simulink model "IEEE14_case"  (R2024b)
settings: Solver=FixedStepAuto  StartTime=0  StopTime=2  FixedStep=1e-7  RelTol=1e-3
values from neighbouring files (symbols this model uses):
  GFL_15_Bva = 0.009    [IEEE14_parameters.m]
  GFL_15_C_bus_pu = 7.179419    [IEEE14_parameters.m]
  GFL_15_f0 = 60    [IEEE14_parameters.m]
  GFL_15_I_id = 691.26967    [IEEE14_parameters.m]
  GFL_15_I_iq = 691.26967    [IEEE14_parameters.m]
  GFL_15_I_od = 45.2207    [IEEE14_parameters.m]
  GFL_15_I_oq = 45.2207    [IEEE14_parameters.m]
  GFL_15_I_pll = 0.78    [IEEE14_parameters.m]
  GFL_15_Kdi = 0.09    [IEEE14_parameters.m]
  GFL_15_Kdo = 0.9    [IEEE14_parameters.m]
  GFL_15_Kqi = 0.09    [IEEE14_parameters.m]
  GFL_15_Kqo = 0.9    [IEEE14_parameters.m]
  GFL_15_Lg_pu = 0.631447    [IEEE14_parameters.m]
  GFL_15_mode = 1    [IEEE14_parameters.m]
  GFL_15_P_id = 3.7166    [IEEE14_parameters.m]
  GFL_15_P_iq = 3.7166    [IEEE14_parameters.m]
  GFL_15_P_od = 0.4798    [IEEE14_parameters.m]
  GFL_15_P_oq = 0.4798    [IEEE14_parameters.m]
  GFL_15_P_pll = 290.42    [IEEE14_parameters.m]
  GFL_15_Qe_ref = 0.2    [IEEE14_parameters.m]
  GFL_15_Rg_pu = 0.024016    [IEEE14_parameters.m]
  GFL_15_Sbase = 1.000000e+4    (= 10000)    [IEEE14_parameters.m]
  GFL_15_Tdi = 0.01    [IEEE14_parameters.m]
  GFL_15_Tdo = 0.2    [IEEE14_parameters.m]
  GFL_15_Tqi = 0.01    [IEEE14_parameters.m]
  GFL_15_Tqo = 0.2    [IEEE14_parameters.m]
  GFL_15_Vbase = 380    [IEEE14_parameters.m]
  GFL_15_Vdc_ref = 1.011475    [IEEE14_parameters.m]
  GFL_15_Vdcbase = 700    [IEEE14_parameters.m]
  GFL_15_vq_ref = 0    [IEEE14_parameters.m]
  GFL_16_Bva = 0.002    [IEEE14_parameters.m]
  GFL_16_C_bus_pu = 7.179419    [IEEE14_parameters.m]
  GFL_16_f0 = 60    [IEEE14_parameters.m]
  GFL_16_I_id = 691.26967    [IEEE14_parameters.m]
  GFL_16_I_iq = 691.26967    [IEEE14_parameters.m]
  GFL_16_I_od = 45.2207    [IEEE14_parameters.m]
  GFL_16_I_oq = 45.2207    [IEEE14_parameters.m]
  GFL_16_I_pll = 0.78    [IEEE14_parameters.m]
  GFL_16_Kdi = 0.05    [IEEE14_parameters.m]
  GFL_16_Kdo = 0.5    [IEEE14_parameters.m]
  GFL_16_Kqi = 0.05    [IEEE14_parameters.m]
  GFL_16_Kqo = 0.5    [IEEE14_parameters.m]
  GFL_16_Lg_pu = 0.631447    [IEEE14_parameters.m]
  GFL_16_mode = 1    [IEEE14_parameters.m]
  GFL_16_P_id = 3.7166    [IEEE14_parameters.m]
  GFL_16_P_iq = 3.7166    [IEEE14_parameters.m]
  GFL_16_P_od = 0.4798    [IEEE14_parameters.m]
  GFL_16_P_oq = 0.4798    [IEEE14_parameters.m]
  GFL_16_P_pll = 290.42    [IEEE14_parameters.m]
  GFL_16_Qe_ref = 0.2    [IEEE14_parameters.m]
  GFL_16_Rg_pu = 0.024016    [IEEE14_parameters.m]
  GFL_16_Sbase = 1.000000e+4    (= 10000)    [IEEE14_parameters.m]
  GFL_16_Tdi = 0.01    [IEEE14_parameters.m]
  GFL_16_Tdo = 0.2    [IEEE14_parameters.m]
  GFL_16_Tqi = 0.01    [IEEE14_parameters.m]
  GFL_16_Tqo = 0.2    [IEEE14_parameters.m]
  GFL_16_Vbase = 380    [IEEE14_parameters.m]
  GFL_16_Vdc_ref = 1.01144    [IEEE14_parameters.m]
  GFL_16_Vdcbase = 700    [IEEE14_parameters.m]
  GFL_16_vq_ref = 0    [IEEE14_parameters.m]
  GFL_17_Bva = 0.002    [IEEE14_parameters.m]
  GFL_17_C_bus_pu = 7.179419    [IEEE14_parameters.m]
  GFL_17_f0 = 60    [IEEE14_parameters.m]
  GFL_17_I_id = 691.26967    [IEEE14_parameters.m]
  GFL_17_I_iq = 691.26967    [IEEE14_parameters.m]
  GFL_17_I_od = 45.2207    [IEEE14_parameters.m]
  GFL_17_I_oq = 45.2207    [IEEE14_parameters.m]
  GFL_17_I_pll = 0.78    [IEEE14_parameters.m]
  GFL_17_Kdi = 0.05    [IEEE14_parameters.m]
  GFL_17_Kdo = 0.5    [IEEE14_parameters.m]
  GFL_17_Kqi = 0.05    [IEEE14_parameters.m]
  GFL_17_Kqo = 0.5    [IEEE14_parameters.m]
  GFL_17_Lg_pu = 0.631447    [IEEE14_parameters.m]
  GFL_17_mode = 1    [IEEE14_parameters.m]
  GFL_17_P_id = 3.7166    [IEEE14_parameters.m]
  GFL_17_P_iq = 3.7166    [IEEE14_parameters.m]
  GFL_17_P_od = 0.4798    [IEEE14_parameters.m]
  GFL_17_P_oq = 0.4798    [IEEE14_parameters.m]
  GFL_17_P_pll = 290.42    [IEEE14_parameters.m]
  GFL_17_Qe_ref = 0.2    [IEEE14_parameters.m]
  GFL_17_Rg_pu = 0.024016    [IEEE14_parameters.m]
  GFL_17_Sbase = 1.000000e+4    (= 10000)    [IEEE14_parameters.m]
  GFL_17_Tdi = 0.01    [IEEE14_parameters.m]
  GFL_17_Tdo = 0.2    [IEEE14_parameters.m]
  GFL_17_Tqi = 0.01    [IEEE14_parameters.m]
  GFL_17_Tqo = 0.2    [IEEE14_parameters.m]
  GFL_17_Vbase = 380    [IEEE14_parameters.m]
  GFL_17_Vdc_ref = 1.011632    [IEEE14_parameters.m]
  GFL_17_Vdcbase = 700    [IEEE14_parameters.m]
  GFL_17_vq_ref = 0    [IEEE14_parameters.m]
  GFL_18_Bva = 0.002    [IEEE14_parameters.m]
  GFL_18_C_bus_pu = 7.179419    [IEEE14_parameters.m]
  GFL_18_f0 = 60    [IEEE14_parameters.m]
  GFL_18_I_id = 691.26967    [IEEE14_parameters.m]
  GFL_18_I_iq = 691.26967    [IEEE14_parameters.m]
  GFL_18_I_od = 45.2207    [IEEE14_parameters.m]
  GFL_18_I_oq = 45.2207    [IEEE14_parameters.m]
  GFL_18_I_pll = 0.78    [IEEE14_parameters.m]
  GFL_18_Kdi = 0.05    [IEEE14_parameters.m]
  GFL_18_Kdo = 0.5    [IEEE14_parameters.m]
  GFL_18_Kqi = 0.05    [IEEE14_parameters.m]
  GFL_18_Kqo = 0.5    [IEEE14_parameters.m]
  GFL_18_Lg_pu = 0.631447    [IEEE14_parameters.m]
  GFL_18_mode = 1    [IEEE14_parameters.m]
  GFL_18_P_id = 3.7166    [IEEE14_parameters.m]
  GFL_18_P_iq = 3.7166    [IEEE14_parameters.m]
  GFL_18_P_od = 0.4798    [IEEE14_parameters.m]
  GFL_18_P_oq = 0.4798    [IEEE14_parameters.m]
  GFL_18_P_pll = 290.42    [IEEE14_parameters.m]
  GFL_18_Qe_ref = 0.2    [IEEE14_parameters.m]
  GFL_18_Rg_pu = 0.024016    [IEEE14_parameters.m]
  GFL_18_Sbase = 1.000000e+4    (= 10000)    [IEEE14_parameters.m]
  GFL_18_Tdi = 0.01    [IEEE14_parameters.m]
  GFL_18_Tdo = 0.2    [IEEE14_parameters.m]
  GFL_18_Tqi = 0.01    [IEEE14_parameters.m]
  GFL_18_Tqo = 0.2    [IEEE14_parameters.m]
  GFL_18_Vbase = 380    [IEEE14_parameters.m]
  GFL_18_Vdc_ref = 1.011572    [IEEE14_parameters.m]
  GFL_18_Vdcbase = 700    [IEEE14_parameters.m]
  GFL_18_vq_ref = 0    [IEEE14_parameters.m]
  ... (+180 more)
(part 2 of 25)

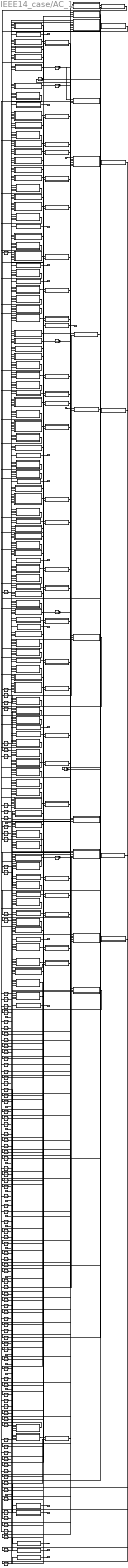
== system IEEE14_case/AC_1 ==
  id_SG_D_1 : Inport
  iq_SG_D_1 : Inport  Port=2
  id_SG_D_2 : Inport  Port=3
  iq_SG_D_2 : Inport  Port=4
  id_SG_D_3 : Inport  Port=5
  iq_SG_D_3 : Inport  Port=6
  id_SG_D_6 : Inport  Port=7
  iq_SG_D_6 : Inport  Port=8
  id_SG_D_8 : Inport  Port=9
  iq_SG_D_8 : Inport  Port=10
  id_GFL_15 : Inport  Port=11
  iq_GFL_15 : Inport  Port=12
  id_GFL_16 : Inport  Port=13
  iq_GFL_16 : Inport  Port=14
  id_GFL_17 : Inport  Port=15
  iq_GFL_17 : Inport  Port=16
  id_GFL_18 : Inport  Port=17
  iq_GFL_18 : Inport  Port=18
  d_id_line_10_11_block : Subsystem
  d_id_line_11_15_block : Subsystem
  d_id_line_12_13_block : Subsystem
  d_id_line_12_16_block : Subsystem
  d_id_line_13_14_block : Subsystem
  d_id_line_13_17_block : Subsystem
  d_id_line_14_18_block : Subsystem
  d_id_line_1_2_block : Subsystem
  d_id_line_1_5_block : Subsystem
  d_id_line_2_3_block : Subsystem
  d_id_line_2_4_block : Subsystem
  d_id_line_2_5_block : Subsystem
  d_id_line_3_4_block : Subsystem
  d_id_line_4_5_block : Subsystem
  d_id_line_4_7_block : Subsystem
  d_id_line_4_9_block : Subsystem
  d_id_line_5_6_block : Subsystem
  d_id_line_6_11_block : Subsystem
  d_id_line_6_12_block : Subsystem
  d_id_line_6_13_block : Subsystem
  d_id_line_7_8_block : Subsystem
  d_id_line_7_9_block : Subsystem
  d_id_line_9_10_block : Subsystem
  d_id_line_9_14_block : Subsystem
  d_id_load_10_block : Subsystem
  d_id_load_11_block : Subsystem
  d_id_load_12_block : Subsystem
  d_id_load_13_block : Subsystem
  d_id_load_14_block : Subsystem
  d_id_load_2_block : Subsystem
  d_id_load_3_block : Subsystem
  d_id_load_4_block : Subsystem
  d_id_load_5_block : Subsystem
  d_id_load_6_block : Subsystem
  d_id_load_9_block : Subsystem
  d_iq_line_10_11_block : Subsystem
  d_iq_line_11_15_block : Subsystem
  d_iq_line_12_13_block : Subsystem
  d_iq_line_12_16_block : Subsystem
  d_iq_line_13_14_block : Subsystem
  d_iq_line_13_17_block : Subsystem
  d_iq_line_14_18_block : Subsystem
  d_iq_line_1_2_block : Subsystem
  d_iq_line_1_5_block : Subsystem
  d_iq_line_2_3_block : Subsystem
  d_iq_line_2_4_block : Subsystem
  d_iq_line_2_5_block : Subsystem
  d_iq_line_3_4_block : Subsystem
  d_iq_line_4_5_block : Subsystem
  d_iq_line_4_7_block : Subsystem
  d_iq_line_4_9_block : Subsystem
  d_iq_line_5_6_block : Subsystem
  d_iq_line_6_11_block : Subsystem
  d_iq_line_6_12_block : Subsystem
  d_iq_line_6_13_block : Subsystem
  d_iq_line_7_8_block : Subsystem
  d_iq_line_7_9_block : Subsystem
  d_iq_line_9_10_block : Subsystem
  d_iq_line_9_14_block : Subsystem
  d_iq_load_10_block : Subsystem
  d_iq_load_11_block : Subsystem
  d_iq_load_12_block : Subsystem
  d_iq_load_13_block : Subsystem
  d_iq_load_14_block : Subsystem
  d_iq_load_2_block : Subsystem
  d_iq_load_3_block : Subsystem
  d_iq_load_4_block : Subsystem
  d_iq_load_5_block : Subsystem
  d_iq_load_6_block : Subsystem
  d_iq_load_9_block : Subsystem
  d_vd_bus_10_block : Subsystem
  d_vd_bus_11_block : Subsystem
  d_vd_bus_12_block : Subsystem
  d_vd_bus_13_block : Subsystem
  d_vd_bus_14_block : Subsystem
  d_vd_bus_15_block : Subsystem
  d_vd_bus_16_block : Subsystem
  d_vd_bus_17_block : Subsystem
  d_vd_bus_18_block : Subsystem
  d_vd_bus_1_block : Subsystem
  d_vd_bus_2_block : Subsystem
  d_vd_bus_3_block : Subsystem
  d_vd_bus_4_block : Subsystem
  d_vd_bus_5_block : Subsystem
  d_vd_bus_6_block : Subsystem
  d_vd_bus_7_block : Subsystem
  d_vd_bus_8_block : Subsystem
  d_vd_bus_9_block : Subsystem
  d_vq_bus_10_block : Subsystem
  d_vq_bus_11_block : Subsystem
  d_vq_bus_12_block : Subsystem
  d_vq_bus_13_block : Subsystem
  d_vq_bus_14_block : Subsystem
  d_vq_bus_15_block : Subsystem
  d_vq_bus_16_block : Subsystem
  d_vq_bus_17_block : Subsystem
  d_vq_bus_18_block : Subsystem
  d_vq_bus_1_block : Subsystem
  d_vq_bus_2_block : Subsystem
  d_vq_bus_3_block : Subsystem
  d_vq_bus_4_block : Subsystem
  d_vq_bus_5_block : Subsystem
  d_vq_bus_6_block : Subsystem
  d_vq_bus_7_block : Subsystem
  d_vq_bus_8_block : Subsystem
  d_vq_bus_9_block : Subsystem
  id_bus_10_block : Subsystem
  id_bus_11_block : Subsystem
  id_bus_12_block : Subsystem
  id_bus_13_block : Subsystem
  id_bus_14_block : Subsystem
  id_bus_15_block : Subsystem
  id_bus_16_block : Subsystem
  id_bus_17_block : Subsystem
  id_bus_18_block : Subsystem
  id_bus_1_block : Subsystem
  id_bus_2_block : Subsystem
  id_bus_3_block : Subsystem
  id_bus_4_block : Subsystem
  id_bus_5_block : Subsystem
  id_bus_6_block : Subsystem
  id_bus_7_block : Subsystem
  id_bus_8_block : Subsystem
  id_bus_9_block : Subsystem
  id_line_10_11 : Integrator  InitialCondition=-0.0994
  id_line_11_15 : Integrator  InitialCondition=-0.0847
  id_line_12_13 : Integrator  InitialCondition=0.0298
  id_line_12_16 : Integrator  InitialCondition=-0.0848
  id_line_13_14 : Integrator  InitialCondition=0.0471
  id_line_13_17 : Integrator  InitialCondition=-0.0854
  id_line_14_18 : Integrator  InitialCondition=-0.0844
  id_line_1_2 : Integrator  InitialCondition=1.2072
  id_line_1_5 : Integrator  InitialCondition=0.5833
  id_line_2_3 : Integrator  InitialCondition=0.6304
  id_line_2_4 : Integrator  InitialCondition=0.4483
  id_line_2_5 : Integrator  InitialCondition=0.3091
  id_line_3_4 : Integrator  InitialCondition=-0.2633
  id_line_4_5 : Integrator  InitialCondition=-0.6044
  id_line_4_7 : Integrator  InitialCondition=0.2064
  id_line_4_9 : Integrator  InitialCondition=0.1163
  id_line_5_6 : Integrator  InitialCondition=0.1823
  id_line_6_11 : Integrator  InitialCondition=0.0515
  id_line_6_12 : Integrator  InitialCondition=0.0172
  id_line_6_13 : Integrator  InitialCondition=0.0733
  id_line_7_8 : Integrator  InitialCondition=-0.0016
  id_line_7_9 : Integrator  InitialCondition=0.1862
  id_line_9_10 : Integrator  InitialCondition=0.0183
  id_line_9_14 : Integrator  InitialCondition=-0.0029
  id_load_10 : Integrator  InitialCondition=0.06873535659071953
  id_load_11 : Integrator  InitialCondition=0.028343117438752577
  id_load_12 : Integrator  InitialCondition=0.05203066731118701
  id_load_13 : Integrator  InitialCondition=0.11216160588057182
  id_load_14 : Integrator  InitialCondition=0.12451829566194553
  id_load_2 : Integrator  InitialCondition=0.19861496427307673
  id_load_3 : Integrator  InitialCondition=0.8795187658248551
  id_load_4 : Integrator  InitialCondition=0.4432908881339787
  id_load_5 : Integrator  InitialCondition=0.06927735163817465
  id_load_6 : Integrator  InitialCondition=0.09154605340717285
  id_load_9 : Integrator  InitialCondition=0.23186808645820936
  iq_bus_10_block : Subsystem
  iq_bus_11_block : Subsystem
  iq_bus_12_block : Subsystem
  iq_bus_13_block : Subsystem
  iq_bus_14_block : Subsystem
  iq_bus_15_block : Subsystem
  iq_bus_16_block : Subsystem
  iq_bus_17_block : Subsystem
  iq_bus_18_block : Subsystem
  iq_bus_1_block : Subsystem
  iq_bus_2_block : Subsystem
  iq_bus_3_block : Subsystem
  iq_bus_4_block : Subsystem
  iq_bus_5_block : Subsystem
  iq_bus_6_block : Subsystem
  iq_bus_7_block : Subsystem
  iq_bus_8_block : Subsystem
  iq_bus_9_block : Subsystem
  iq_line_10_11 : Integrator  InitialCondition=-0.0778
  iq_line_11_15 : Integrator  InitialCondition=0.0403
  iq_line_12_13 : Integrator  InitialCondition=-0.0166
  iq_line_12_16 : Integrator  InitialCondition=0.0398
  iq_line_13_14 : Integrator  InitialCondition=0.0205
  iq_line_13_17 : Integrator  InitialCondition=0.0402
  iq_line_14_18 : Integrator  InitialCondition=0.0417
  iq_line_1_2 : Integrator  InitialCondition=0.0983
  iq_line_1_5 : Integrator  InitialCondition=0.0958
  iq_line_2_3 : Integrator  InitialCondition=-0.1082
  iq_line_2_4 : Integrator  InitialCondition=0.1344
  iq_line_2_5 : Integrator  InitialCondition=0.1439
  iq_line_3_4 : Integrator  InitialCondition=0.1816
  iq_line_4_5 : Integrator  InitialCondition=0.0405
  iq_line_4_7 : Integrator  InitialCondition=0.1587
  iq_line_4_9 : Integrator  InitialCondition=0.0708
  iq_line_5_6 : Integrator  InitialCondition=0.0222
  iq_line_6_11 : Integrator  InitialCondition=0.1413
  iq_line_6_12 : Integrator  InitialCondition=0.11
  iq_line_6_13 : Integrator  InitialCondition=0.1609
  iq_line_7_8 : Integrator  InitialCondition=-0.0082
  iq_line_7_9 : Integrator  InitialCondition=0.0516
  iq_line_9_10 : Integrator  InitialCondition=0.0881
  iq_line_9_14 : Integrator  InitialCondition=-0.0308
  iq_load_10 : Integrator  InitialCondition=-0.06784560660059201
  iq_load_11 : Integrator  InitialCondition=-0.021996168279197863
  iq_load_12 : Integrator  InitialCondition=-0.02423326671806508
  iq_load_13 : Integrator  InitialCondition=-0.0749088369050284
  iq_load_14 : Integrator  InitialCondition=-0.07210105053188964
  iq_load_2 : Integrator  InitialCondition=-0.13580394701233528
  iq_load_3 : Integrator  InitialCondition=-0.3629254076686232
  iq_load_4 : Integrator  InitialCondition=-0.10576972487588117
  iq_load_5 : Integrator  InitialCondition=-0.02416665828239703
  iq_load_6 : Integrator  InitialCondition=-0.0865380168455866
  iq_load_9 : Integrator  InitialCondition=-0.20188514867386012
  vd_bus_1 : Integrator  InitialCondition=1.06
  vd_bus_10 : Integrator  InitialCondition=1.0850866003154533
  vd_bus_11 : Integrator  InitialCondition=1.0782933921318274
  vd_bus_12 : Integrator  InitialCondition=1.0810945989476521
  vd_bus_13 : Integrator  InitialCondition=1.0711851912075123
  vd_bus_14 : Integrator  InitialCondition=1.0702741301344978
  vd_bus_15 : Integrator  InitialCondition=1.1116110968480268
  vd_bus_15_out_block : Subsystem
  vd_bus_16 : Integrator  InitialCondition=1.11407591885913
  vd_bus_16_out_block : Subsystem
  vd_bus_17 : Integrator  InitialCondition=1.1044709003041506
  vd_bus_17_out_block : Subsystem
  vd_bus_18 : Integrator  InitialCondition=1.1045577407027038
  vd_bus_18_out_block : Subsystem
  vd_bus_1_out_block : Subsystem
  vd_bus_2 : Integrator  InitialCondition=1.0424236711882215
  vd_bus_2_out_block : Subsystem
  vd_bus_3 : Integrator  InitialCondition=0.9913775753162218
  vd_bus_3_out_block : Subsystem
  vd_bus_4 : Integrator  InitialCondition=1.040078267757068
  vd_bus_5 : Integrator  InitialCondition=1.0498509288179132
  vd_bus_6 : Integrator  InitialCondition=1.055074232738516
  vd_bus_6_out_block : Subsystem
  vd_bus_7 : Integrator  InitialCondition=1.072545462130714
  vd_bus_8 : Integrator  InitialCondition=1.0710963964517566
  vd_bus_8_out_block : Subsystem
  vd_bus_9 : Integrator  InitialCondition=1.0782222211377726
  vq_bus_1 : Integrator  InitialCondition=0.0
  vq_bus_10 : Integrator  InitialCondition=-0.22722452297111975
  vq_bus_11 : Integrator  InitialCondition=-0.2017534916558011
  vq_bus_12 : Integrator  InitialCondition=-0.19600851364759078
  vq_bus_13 : Integrator  InitialCondition=-0.19829634756591635
  vq_bus_14 : Integrator  InitialCondition=-0.21818391422220956
  vq_bus_15 : Integrator  InitialCondition=-0.1448821101871742
  vq_bus_15_out_block : Subsystem
  vq_bus_16 : Integrator  InitialCondition=-0.13904857608995075
  vq_bus_16_out_block : Subsystem
  vq_bus_17 : Integrator  InitialCondition=-0.140924628484122
  vq_bus_17_out_block : Subsystem
  vq_bus_18 : Integrator  InitialCondition=-0.16158890681408472
  vq_bus_18_out_block : Subsystem
  vq_bus_1_out_block : Subsystem
  vq_bus_2 : Integrator  InitialCondition=-0.07333409675226385
  vq_bus_2_out_block : Subsystem
  vq_bus_3 : Integrator  InitialCondition=-0.1930556996312955
  vq_bus_3_out_block : Subsystem
  vq_bus_4 : Integrator  InitialCondition=-0.1601855443701038
  vq_bus_5 : Integrator  InitialCondition=-0.13527348292909663
  vq_bus_6 : Integrator  InitialCondition=-0.17809650027788754
  vq_bus_6_out_block : Subsystem
  vq_bus_7 : Integrator  InitialCondition=-0.20239348167849394
  vq_bus_8 : Integrator  InitialCondition=-0.20212003737398646
  vq_bus_8_out_block : Subsystem
  vq_bus_9 : Integrator  InitialCondition=-0.22287264369679838
  vd_bus_1_out : Outport
  vq_bus_1_out : Outport  Port=2
  vd_bus_2_out : Outport  Port=3
  vq_bus_2_out : Outport  Port=4
  vd_bus_3_out : Outport  Port=5
  vq_bus_3_out : Outport  Port=6
  vd_bus_6_out : Outport  Port=7
  vq_bus_6_out : Outport  Port=8
  vd_bus_8_out : Outport  Port=9
  vq_bus_8_out : Outport  Port=10
  vd_bus_15_out : Outport  Port=11
  vq_bus_15_out : Outport  Port=12
  vd_bus_16_out : Outport  Port=13
  vq_bus_16_out : Outport  Port=14
  vd_bus_17_out : Outport  Port=15
  vq_bus_17_out : Outport  Port=16
  vd_bus_18_out : Outport  Port=17
  vq_bus_18_out : Outport  Port=18
  wires:
  d_id_load_12_block/1(Blockout_d_id_load_12_58f44) -> id_load_12/1
  vd_bus_8/1 -> vd_bus_8_out_block/1(State_vd_bus_8_bc007), d_id_line_7_8_block/3(State_vd_bus_8_dd54f), d_vq_bus_8_block/2(State_vd_bus_8_3801a)
  vq_bus_16_out_block/1(Blockout_vq_bus_16_out_7f446) -> vq_bus_16_out/1
  d_vq_bus_11_block/1(Blockout_d_vq_bus_11_d741b) -> vq_bus_11/1
  id_GFL_15/1 -> id_bus_15_block/1(Input_id_GFL_15_c7559)
  d_id_line_9_14_block/1(Blockout_d_id_line_9_14_6ccdc) -> id_line_9_14/1
  iq_GFL_17/1 -> iq_bus_17_block/1(Input_iq_GFL_17_ce0cb)
  d_id_line_6_12_block/1(Blockout_d_id_line_6_12_9a391) -> id_line_6_12/1
  iq_GFL_18/1 -> iq_bus_18_block/1(Input_iq_GFL_18_ec44c)
  id_line_12_16/1 -> d_id_line_12_16_block/1(State_id_line_12_16_7c285), d_iq_line_12_16_block/1(State_id_line_12_16_8add4), id_bus_16_block/2(State_id_line_12_16_7c95c), id_bus_12_block/4(State_id_line_12_16_716c0)
  iq_bus_6_block/1(Blockout_iq_bus_6_4d630) -> d_vq_bus_6_block/1(Alge_iq_bus_6_86836)
  d_vq_bus_15_block/1(Blockout_d_vq_bus_15_3c6af) -> vq_bus_15/1
  id_load_10/1 -> d_id_load_10_block/1(State_id_load_10_31e9c), d_iq_load_10_block/1(State_id_load_10_0a094), id_bus_10_block/1(State_id_load_10_5dfe0)
  id_line_7_8/1 -> d_iq_line_7_8_block/1(State_id_line_7_8_32461), id_bus_7_block/2(State_id_line_7_8_a9fc4), id_bus_8_block/2(State_id_line_7_8_1f3e4)
  id_SG_D_2/1 -> id_bus_2_block/1(Input_id_SG_D_2_87b72)
  iq_line_4_5/1 -> iq_bus_4_block/4(State_iq_line_4_5_4a221), iq_bus_5_block/4(State_iq_line_4_5_98539), d_id_line_4_5_block/2(State_iq_line_4_5_5f8a8), d_iq_line_4_5_block/2(State_iq_line_4_5_0332d)
  d_id_line_7_9_block/1(Blockout_d_id_line_7_9_bf772) -> id_line_7_9/1
  id_bus_8_block/1(Blockout_id_bus_8_d2e4f) -> d_vd_bus_8_block/1(Alge_id_bus_8_67a63)
  vq_bus_2/1 -> d_vd_bus_2_block/2(State_vq_bus_2_bcae6), d_iq_line_1_2_block/4(State_vq_bus_2_0b7a1), d_iq_line_2_5_block/3(State_vq_bus_2_080ca), d_iq_line_2_4_block/3(State_vq_bus_2_24316), d_iq_load_2_block/3(State_vq_bus_2_25b3a), vq_bus_2_out_block/1(State_vq_bus_2_ea0d1), d_iq_line_2_3_block/3(State_vq_bus_2_4a159)
  id_GFL_18/1 -> id_bus_18_block/1(Input_id_GFL_18_1db57)
  d_vq_bus_12_block/1(Blockout_d_vq_bus_12_08cfc) -> vq_bus_12/1
  id_bus_13_block/1(Blockout_id_bus_13_73688) -> d_vd_bus_13_block/1(Alge_id_bus_13_3078a)
  iq_bus_16_block/1(Blockout_iq_bus_16_71499) -> d_vq_bus_16_block/1(Alge_iq_bus_16_45d99)
  iq_line_12_16/1 -> d_iq_line_12_16_block/2(State_iq_line_12_16_8bc6b), iq_bus_12_block/4(State_iq_line_12_16_8cacc), iq_bus_16_block/2(State_iq_line_12_16_2996d), d_id_line_12_16_block/2(State_iq_line_12_16_b3649)
  d_iq_load_12_block/1(Blockout_d_iq_load_12_9f109) -> iq_load_12/1
  d_iq_line_4_5_block/1(Blockout_d_iq_line_4_5_de0fa) -> iq_line_4_5/1
  d_id_line_10_11_block/1(Blockout_d_id_line_10_11_2eb24) -> id_line_10_11/1
  vd_bus_16_out_block/1(Blockout_vd_bus_16_out_bf920) -> vd_bus_16_out/1
  id_GFL_16/1 -> id_bus_16_block/1(Input_id_GFL_16_67778)
  id_GFL_17/1 -> id_bus_17_block/1(Input_id_GFL_17_1404c)
  vd_bus_14/1 -> d_id_load_14_block/3(State_vd_bus_14_a8c17), d_id_line_14_18_block/3(State_vd_bus_14_f98b2), d_id_line_9_14_block/3(State_vd_bus_14_60cbb), d_vq_bus_14_block/2(State_vd_bus_14_b82c6), d_id_line_13_14_block/4(State_vd_bus_14_db328)
  iq_line_6_11/1 -> iq_bus_6_block/4(State_iq_line_6_11_dc417), iq_bus_11_block/2(State_iq_line_6_11_3bc55), d_id_line_6_11_block/2(State_iq_line_6_11_43c10), d_iq_line_6_11_block/2(State_iq_line_6_11_23688)
  iq_SG_D_3/1 -> iq_bus_3_block/1(Input_iq_SG_D_3_f2caf)
  d_id_load_14_block/1(Blockout_d_id_load_14_efc39) -> id_load_14/1
  id_line_2_3/1 -> id_bus_2_block/4(State_id_line_2_3_47528), id_bus_3_block/3(State_id_line_2_3_0c1e5), d_iq_line_2_3_block/1(State_id_line_2_3_74cbb), d_id_line_2_3_block/1(State_id_line_2_3_bbe6e)
  iq_GFL_15/1 -> iq_bus_15_block/1(Input_iq_GFL_15_581cf)
  iq_GFL_16/1 -> iq_bus_16_block/1(Input_iq_GFL_16_66c6c)
  d_id_line_9_10_block/1(Blockout_d_id_line_9_10_ec156) -> id_line_9_10/1
  vd_bus_4/1 -> d_id_line_2_4_block/4(State_vd_bus_4_3c016), d_id_line_4_5_block/3(State_vd_bus_4_6b1ed), d_id_line_4_7_block/2(State_vd_bus_4_7fac7), d_id_load_4_block/3(State_vd_bus_4_11e1c), d_id_line_4_9_block/2(State_vd_bus_4_34e3c), d_id_line_3_4_block/4(State_vd_bus_4_4b57b), d_vq_bus_4_block/2(State_vd_bus_4_7baed)
  id_bus_18_block/1(Blockout_id_bus_18_37cb9) -> d_vd_bus_18_block/1(Alge_id_bus_18_48e95)
  id_bus_9_block/1(Blockout_id_bus_9_1c066) -> d_vd_bus_9_block/1(Alge_id_bus_9_e9a9d)
  iq_load_9/1 -> d_id_load_9_block/2(State_iq_load_9_3ccc7), iq_bus_9_block/1(State_iq_load_9_b0a53), d_iq_load_9_block/2(State_iq_load_9_3e6fb)
  iq_bus_9_block/1(Blockout_iq_bus_9_d3dd5) -> d_vq_bus_9_block/1(Alge_iq_bus_9_5db18)
  d_iq_line_11_15_block/1(Blockout_d_iq_line_11_15_665a1) -> iq_line_11_15/1
  iq_line_7_8/1 -> iq_bus_8_block/2(State_iq_line_7_8_02a2e), iq_bus_7_block/2(State_iq_line_7_8_54428), d_id_line_7_8_block/1(State_iq_line_7_8_7266b)
  vd_bus_15_out_block/1(Blockout_vd_bus_15_out_53236) -> vd_bus_15_out/1
  vq_bus_18/1 -> d_vd_bus_18_block/2(State_vq_bus_18_c75a6), d_iq_line_14_18_block/4(State_vq_bus_18_e3293), vq_bus_18_out_block/1(State_vq_bus_18_e31db)
  iq_SG_D_6/1 -> iq_bus_6_block/1(Input_iq_SG_D_6_fd9b5)
  iq_SG_D_8/1 -> iq_bus_8_block/1(Input_iq_SG_D_8_05cc5)
  vd_bus_18_out_block/1(Blockout_vd_bus_18_out_c2e2f) -> vd_bus_18_out/1
  id_load_5/1 -> id_bus_5_block/1(State_id_load_5_1b867), d_iq_load_5_block/1(State_id_load_5_e43f2), d_id_load_5_block/1(State_id_load_5_82a6e)
  vq_bus_12/1 -> d_vd_bus_12_block/2(State_vq_bus_12_ee0ac), d_iq_line_12_16_block/3(State_vq_bus_12_58935), d_iq_load_12_block/3(State_vq_bus_12_83802), d_iq_line_12_13_block/3(State_vq_bus_12_5dc3a), d_iq_line_6_12_block/3(State_vq_bus_12_69550)
  id_SG_D_8/1 -> id_bus_8_block/1(Input_id_SG_D_8_15cec)
  d_id_load_11_block/1(Blockout_d_id_load_11_86202) -> id_load_11/1
  vq_bus_17/1 -> d_vd_bus_17_block/2(State_vq_bus_17_647a1), d_iq_line_13_17_block/4(State_vq_bus_17_e9502), vq_bus_17_out_block/1(State_vq_bus_17_ceb31)
  iq_bus_18_block/1(Blockout_iq_bus_18_97ded) -> d_vq_bus_18_block/1(Alge_iq_bus_18_569e7)
  iq_line_6_12/1 -> d_id_line_6_12_block/2(State_iq_line_6_12_68573), iq_bus_6_block/5(State_iq_line_6_12_b02a7), iq_bus_12_block/2(State_iq_line_6_12_a1863), d_iq_line_6_12_block/2(State_iq_line_6_12_950d7)
  id_SG_D_3/1 -> id_bus_3_block/1(Input_id_SG_D_3_ffe04)
  id_SG_D_6/1 -> id_bus_6_block/1(Input_id_SG_D_6_e5cad)
  iq_bus_1_block/1(Blockout_iq_bus_1_352cb) -> d_vq_bus_1_block/1(Alge_iq_bus_1_7f6e6)
  iq_SG_D_2/1 -> iq_bus_2_block/1(Input_iq_SG_D_2_8fd05)
  vd_bus_1/1 -> d_vq_bus_1_block/2(State_vd_bus_1_cd54b), vd_bus_1_out_block/1(State_vd_bus_1_5dc0e), d_id_line_1_5_block/3(State_vd_bus_1_768e4), d_id_line_1_2_block/3(State_vd_bus_1_70d37)
  id_bus_17_block/1(Blockout_id_bus_17_789d1) -> d_vd_bus_17_block/1(Alge_id_bus_17_262b4)
  vq_bus_2_out_block/1(Blockout_vq_bus_2_out_c2eb9) -> vq_bus_2_out/1
  vd_bus_6/1 -> d_vq_bus_6_block/2(State_vd_bus_6_d464c), d_id_load_6_block/3(State_vd_bus_6_858b4), d_id_line_6_12_block/4(State_vd_bus_6_ffde5), d_id_line_6_13_block/4(State_vd_bus_6_845eb), vd_bus_6_out_block/1(State_vd_bus_6_a4f60), d_id_line_5_6_block/3(State_vd_bus_6_a8e09), d_id_line_6_11_block/4(State_vd_bus_6_98960)
  d_vd_bus_18_block/1(Blockout_d_vd_bus_18_49967) -> vd_bus_18/1
  iq_SG_D_1/1 -> iq_bus_1_block/1(Input_iq_SG_D_1_56ece)
  iq_line_2_5/1 -> iq_bus_5_block/3(State_iq_line_2_5_08804), d_id_line_2_5_block/2(State_iq_line_2_5_b0efa), iq_bus_2_block/6(State_iq_line_2_5_fb0c4), d_iq_line_2_5_block/2(State_iq_line_2_5_dd836)
  iq_bus_3_block/1(Blockout_iq_bus_3_60c7d) -> d_vq_bus_3_block/1(Alge_iq_bus_3_8efd3)
  id_SG_D_1/1 -> id_bus_1_block/1(Input_id_SG_D_1_3327d)
  id_bus_1_block/1(Blockout_id_bus_1_ba05b) -> d_vd_bus_1_block/1(Alge_id_bus_1_90b3c)
  vd_bus_7/1 -> d_vq_bus_7_block/2(State_vd_bus_7_1c88a), d_id_line_4_7_block/3(State_vd_bus_7_4017f), d_id_line_7_9_block/2(State_vd_bus_7_8bd9d), d_id_line_7_8_block/2(State_vd_bus_7_8b12e)
  d_vq_bus_4_block/1(Blockout_d_vq_bus_4_75eba) -> vq_bus_4/1
  vd_bus_16/1 -> d_vq_bus_16_block/2(State_vd_bus_16_358d8), d_id_line_12_16_block/4(State_vd_bus_16_b2ca7), vd_bus_16_out_block/1(State_vd_bus_16_c68f5)
  id_bus_5_block/1(Blockout_id_bus_5_9fe33) -> d_vd_bus_5_block/1(Alge_id_bus_5_3a39c)
  iq_line_9_10/1 -> d_id_line_9_10_block/2(State_iq_line_9_10_22e13), d_iq_line_9_10_block/2(State_iq_line_9_10_78cd2), iq_bus_9_block/4(State_iq_line_9_10_294ee), iq_bus_10_block/2(State_iq_line_9_10_4cded)
  d_iq_line_7_8_block/1(Blockout_d_iq_line_7_8_a0a04) -> iq_line_7_8/1
  vq_bus_15/1 -> d_vd_bus_15_block/2(State_vq_bus_15_3aaea), d_iq_line_11_15_block/4(State_vq_bus_15_132fc), vq_bus_15_out_block/1(State_vq_bus_15_e85b0)
  iq_bus_17_block/1(Blockout_iq_bus_17_2a23f) -> d_vq_bus_17_block/1(Alge_iq_bus_17_e020e)
  vd_bus_13/1 -> d_vq_bus_13_block/2(State_vd_bus_13_68df6), d_id_line_6_13_block/3(State_vd_bus_13_13060), d_id_line_13_14_block/3(State_vd_bus_13_a4a43), d_id_line_12_13_block/4(State_vd_bus_13_1a95e), d_id_load_13_block/3(State_vd_bus_13_31285), d_id_line_13_17_block/3(State_vd_bus_13_e5c14)
  vd_bus_10/1 -> d_id_line_9_10_block/3(State_vd_bus_10_33748), d_id_load_10_block/3(State_vd_bus_10_d1446), d_id_line_10_11_block/3(State_vd_bus_10_b9381), d_vq_bus_10_block/2(State_vd_bus_10_4ea61)
  id_bus_10_block/1(Blockout_id_bus_10_ed934) -> d_vd_bus_10_block/1(Alge_id_bus_10_8b36b)
  id_line_9_10/1 -> d_id_line_9_10_block/1(State_id_line_9_10_959cd), d_iq_line_9_10_block/1(State_id_line_9_10_7d192), id_bus_10_block/2(State_id_line_9_10_2483c), id_bus_9_block/4(State_id_line_9_10_faf7e)
  vq_bus_15_out_block/1(Blockout_vq_bus_15_out_b5487) -> vq_bus_15_out/1
  iq_bus_4_block/1(Blockout_iq_bus_4_8bc6d) -> d_vq_bus_4_block/1(Alge_iq_bus_4_ff8e3)
  id_bus_16_block/1(Blockout_id_bus_16_bdc3f) -> d_vd_bus_16_block/1(Alge_id_bus_16_8d52e)
  vq_bus_9/1 -> d_iq_line_4_9_block/3(State_vq_bus_9_e7de0), d_iq_line_7_9_block/3(State_vq_bus_9_3c7a5), d_iq_line_9_14_block/4(State_vq_bus_9_d4758), d_iq_load_9_block/3(State_vq_bus_9_1c480), d_vd_bus_9_block/2(State_vq_bus_9_42a9a), d_iq_line_9_10_block/4(State_vq_bus_9_d6463)
  id_bus_15_block/1(Blockout_id_bus_15_e9971) -> d_vd_bus_15_block/1(Alge_id_bus_15_fd09e)
  id_bus_6_block/1(Blockout_id_bus_6_5cca2) -> d_vd_bus_6_block/1(Alge_id_bus_6_e431e)
  d_id_line_2_5_block/1(Blockout_d_id_line_2_5_7bd8a) -> id_line_2_5/1
  id_line_3_4/1 -> id_bus_3_block/4(State_id_line_3_4_0527c), id_bus_4_block/3(State_id_line_3_4_6920e), d_iq_line_3_4_block/1(State_id_line_3_4_7c07a), d_id_line_3_4_block/1(State_id_line_3_4_8ed23)
  iq_bus_15_block/1(Blockout_iq_bus_15_665d9) -> d_vq_bus_15_block/1(Alge_iq_bus_15_82ed5)
  d_iq_line_6_11_block/1(Blockout_d_iq_line_6_11_ea354) -> iq_line_6_11/1
  iq_line_11_15/1 -> d_id_line_11_15_block/2(State_iq_line_11_15_e6608), d_iq_line_11_15_block/2(State_iq_line_11_15_b5696), iq_bus_15_block/2(State_iq_line_11_15_dae91), iq_bus_11_block/4(State_iq_line_11_15_05d46)
  iq_line_13_17/1 -> d_id_line_13_17_block/2(State_iq_line_13_17_a0741), iq_bus_17_block/2(State_iq_line_13_17_ac3bf), d_iq_line_13_17_block/2(State_iq_line_13_17_7cac6), iq_bus_13_block/5(State_iq_line_13_17_718e0)
  id_line_12_13/1 -> d_id_line_12_13_block/1(State_id_line_12_13_dd6c1), id_bus_12_block/3(State_id_line_12_13_b0c21), d_iq_line_12_13_block/1(State_id_line_12_13_b8b65), id_bus_13_block/3(State_id_line_12_13_8b355)
  iq_bus_14_block/1(Blockout_iq_bus_14_9d2f8) -> d_vq_bus_14_block/1(Alge_iq_bus_14_0b3bc)
  id_bus_14_block/1(Blockout_id_bus_14_6847e) -> d_vd_bus_14_block/1(Alge_id_bus_14_7a3c0)
  vd_bus_2_out_block/1(Blockout_vd_bus_2_out_d1efc) -> vd_bus_2_out/1
  id_bus_3_block/1(Blockout_id_bus_3_cecd1) -> d_vd_bus_3_block/1(Alge_id_bus_3_b82db)
  iq_bus_13_block/1(Blockout_iq_bus_13_89032) -> d_vq_bus_13_block/1(Alge_iq_bus_13_d5ed4)
  iq_bus_7_block/1(Blockout_iq_bus_7_85d72) -> d_vq_bus_7_block/1(Alge_iq_bus_7_36c94)
  iq_bus_12_block/1(Blockout_iq_bus_12_5a9dd) -> d_vq_bus_12_block/1(Alge_iq_bus_12_a824a)
  iq_bus_11_block/1(Blockout_iq_bus_11_5f78a) -> d_vq_bus_11_block/1(Alge_iq_bus_11_f813e)
  id_bus_12_block/1(Blockout_id_bus_12_1147b) -> d_vd_bus_12_block/1(Alge_id_bus_12_768d8)
  id_bus_11_block/1(Blockout_id_bus_11_f1534) -> d_vd_bus_11_block/1(Alge_id_bus_11_fad28)
  vd_bus_17/1 -> d_vq_bus_17_block/2(State_vd_bus_17_c4074), d_id_line_13_17_block/4(State_vd_bus_17_94433), vd_bus_17_out_block/1(State_vd_bus_17_d959d)
  iq_bus_10_block/1(Blockout_iq_bus_10_4d9cc) -> d_vq_bus_10_block/1(Alge_iq_bus_10_83323)
  iq_line_2_3/1 -> d_id_line_2_3_block/2(State_iq_line_2_3_6cbab), d_iq_line_2_3_block/2(State_iq_line_2_3_6a30b), iq_bus_3_block/3(State_iq_line_2_3_b53b7), iq_bus_2_block/4(State_iq_line_2_3_ceafd)
  iq_load_11/1 -> iq_bus_11_block/1(State_iq_load_11_c9523), d_iq_load_11_block/2(State_iq_load_11_f52d6), d_id_load_11_block/2(State_iq_load_11_d9a12)
  iq_line_10_11/1 -> d_id_line_10_11_block/2(State_iq_line_10_11_98837), d_iq_line_10_11_block/2(State_iq_line_10_11_0ead8), iq_bus_11_block/3(State_iq_line_10_11_5b2aa), iq_bus_10_block/3(State_iq_line_10_11_32883)
  iq_bus_8_block/1(Blockout_iq_bus_8_a9e89) -> d_vq_bus_8_block/1(Alge_iq_bus_8_97cc9)
  id_line_11_15/1 -> d_iq_line_11_15_block/1(State_id_line_11_15_35576), id_bus_15_block/2(State_id_line_11_15_010a9), id_bus_11_block/4(State_id_line_11_15_2f637), d_id_line_11_15_block/1(State_id_line_11_15_bc21e)
  id_bus_7_block/1(Blockout_id_bus_7_ec462) -> d_vd_bus_7_block/1(Alge_id_bus_7_a7561)
  d_vd_bus_7_block/1(Blockout_d_vd_bus_7_1c15c) -> vd_bus_7/1
  iq_bus_5_block/1(Blockout_iq_bus_5_f0651) -> d_vq_bus_5_block/1(Alge_iq_bus_5_baf50)
  iq_load_5/1 -> iq_bus_5_block/1(State_iq_load_5_72501), d_iq_load_5_block/2(State_iq_load_5_ed9b4), d_id_load_5_block/2(State_iq_load_5_f0bf8)
  iq_line_5_6/1 -> iq_bus_5_block/5(State_iq_line_5_6_789df), d_id_line_5_6_block/1(State_iq_line_5_6_d8c49), iq_bus_6_block/3(State_iq_line_5_6_4236b)
  id_bus_4_block/1(Blockout_id_bus_4_5067c) -> d_vd_bus_4_block/1(Alge_id_bus_4_f94e7)
  d_id_line_7_8_block/1(Blockout_d_id_line_7_8_3aa11) -> id_line_7_8/1
  vq_bus_8_out_block/1(Blockout_vq_bus_8_out_36371) -> vq_bus_8_out/1
  vd_bus_3/1 -> d_vq_bus_3_block/2(State_vd_bus_3_9f628), d_id_load_3_block/3(State_vd_bus_3_b5bb0), d_id_line_2_3_block/4(State_vd_bus_3_a3e95), vd_bus_3_out_block/1(State_vd_bus_3_4d21d), d_id_line_3_4_block/3(State_vd_bus_3_4e043)
  iq_bus_2_block/1(Blockout_iq_bus_2_d0264) -> d_vq_bus_2_block/1(Alge_iq_bus_2_c94ee)
  id_bus_2_block/1(Blockout_id_bus_2_89082) -> d_vd_bus_2_block/1(Alge_id_bus_2_b20cd)
  vq_bus_18_out_block/1(Blockout_vq_bus_18_out_45376) -> vq_bus_18_out/1
  d_iq_load_9_block/1(Blockout_d_iq_load_9_c9e01) -> iq_load_9/1
  d_id_line_1_2_block/1(Blockout_d_id_line_1_2_e6d8f) -> id_line_1_2/1
  vq_bus_17_out_block/1(Blockout_vq_bus_17_out_c5b42) -> vq_bus_17_out/1
  id_line_6_13/1 -> id_bus_6_block/6(State_id_line_6_13_76e25), d_iq_line_6_13_block/1(State_id_line_6_13_f1d85), id_bus_13_block/2(State_id_line_6_13_33910), d_id_line_6_13_block/1(State_id_line_6_13_e3fb9)
  d_id_load_3_block/1(Blockout_d_id_load_3_c7879) -> id_load_3/1
  vd_bus_17_out_block/1(Blockout_vd_bus_17_out_ee528) -> vd_bus_17_out/1
  vd_bus_8_out_block/1(Blockout_vd_bus_8_out_d3476) -> vd_bus_8_out/1
  vd_bus_11/1 -> d_id_line_6_11_block/3(State_vd_bus_11_0f741), d_vq_bus_11_block/2(State_vd_bus_11_1dc97), d_id_line_10_11_block/4(State_vd_bus_11_0464d), d_id_line_11_15_block/3(State_vd_bus_11_d33d1), d_id_load_11_block/3(State_vd_bus_11_633a4)
  d_iq_line_3_4_block/1(Blockout_d_iq_line_3_4_fcd14) -> iq_line_3_4/1
  vq_bus_6_out_block/1(Blockout_vq_bus_6_out_b9abb) -> vq_bus_6_out/1
  d_iq_load_2_block/1(Blockout_d_iq_load_2_9dea5) -> iq_load_2/1
  vd_bus_6_out_block/1(Blockout_vd_bus_6_out_fb39e) -> vd_bus_6_out/1
  vq_bus_3_out_block/1(Blockout_vq_bus_3_out_bf333) -> vq_bus_3_out/1
  id_load_9/1 -> id_bus_9_block/1(State_id_load_9_3577c), d_id_load_9_block/1(State_id_load_9_8af8e), d_iq_load_9_block/1(State_id_load_9_c0f8a)
  vd_bus_3_out_block/1(Blockout_vd_bus_3_out_e3de8) -> vd_bus_3_out/1
  vq_bus_3/1 -> d_iq_load_3_block/3(State_vq_bus_3_60dd0), d_iq_line_2_3_block/4(State_vq_bus_3_fc550), vq_bus_3_out_block/1(State_vq_bus_3_c1e3e), d_vd_bus_3_block/2(State_vq_bus_3_fe7bf), d_iq_line_3_4_block/3(State_vq_bus_3_c19a2)
  vq_bus_1_out_block/1(Blockout_vq_bus_1_out_08423) -> vq_bus_1_out/1
  id_line_2_4/1 -> id_bus_4_block/2(State_id_line_2_4_71476), id_bus_2_block/5(State_id_line_2_4_54727), d_iq_line_2_4_block/1(State_id_line_2_4_5b6e3), d_id_line_2_4_block/1(State_id_line_2_4_e6465)
  id_line_13_14/1 -> id_bus_14_block/3(State_id_line_13_14_e8dab), id_bus_13_block/4(State_id_line_13_14_d0ea7), d_iq_line_13_14_block/1(State_id_line_13_14_fcef8), d_id_line_13_14_block/1(State_id_line_13_14_79a4b)
  iq_line_4_9/1 -> d_id_line_4_9_block/1(State_iq_line_4_9_4287b), iq_bus_9_block/2(State_iq_line_4_9_4d417), iq_bus_4_block/6(State_iq_line_4_9_e8dca)
  vd_bus_1_out_block/1(Blockout_vd_bus_1_out_41eef) -> vd_bus_1_out/1
  d_id_line_14_18_block/1(Blockout_d_id_line_14_18_3e263) -> id_line_14_18/1
  id_line_2_5/1 -> d_id_line_2_5_block/1(State_id_line_2_5_d145b), id_bus_5_block/3(State_id_line_2_5_8adac), id_bus_2_block/6(State_id_line_2_5_398b7), d_iq_line_2_5_block/1(State_id_line_2_5_ba290)
  d_id_line_13_17_block/1(Blockout_d_id_line_13_17_24730) -> id_line_13_17/1
  d_iq_line_12_16_block/1(Blockout_d_iq_line_12_16_95ad9) -> iq_line_12_16/1
  vq_bus_1/1 -> d_vd_bus_1_block/2(State_vq_bus_1_8d526), d_iq_line_1_2_block/3(State_vq_bus_1_f6968), d_iq_line_1_5_block/3(State_vq_bus_1_1731e), vq_bus_1_out_block/1(State_vq_bus_1_00178)
  iq_load_2/1 -> d_id_load_2_block/2(State_iq_load_2_a0763), iq_bus_2_block/2(State_iq_load_2_0a4eb), d_iq_load_2_block/2(State_iq_load_2_39818)
  iq_line_4_7/1 -> d_id_line_4_7_block/1(State_iq_line_4_7_27056), iq_bus_7_block/1(State_iq_line_4_7_bfb83), iq_bus_4_block/5(State_iq_line_4_7_17bcc)
  vq_bus_16/1 -> d_vd_bus_16_block/2(State_vq_bus_16_21a55), d_iq_line_12_16_block/4(State_vq_bus_16_f8d4f), vq_bus_16_out_block/1(State_vq_bus_16_bbd15)
  iq_line_6_13/1 -> d_id_line_6_13_block/2(State_iq_line_6_13_c66be), d_iq_line_6_13_block/2(State_iq_line_6_13_f7b4b), iq_bus_13_block/2(State_iq_line_6_13_f63e3), iq_bus_6_block/6(State_iq_line_6_13_efd13)
  id_line_14_18/1 -> d_id_line_14_18_block/1(State_id_line_14_18_fb6d6), d_iq_line_14_18_block/1(State_id_line_14_18_708e0), id_bus_14_block/4(State_id_line_14_18_ae0a4), id_bus_18_block/2(State_id_line_14_18_0ac94)
  d_iq_line_10_11_block/1(Blockout_d_iq_line_10_11_8dcae) -> iq_line_10_11/1
  d_id_line_6_13_block/1(Blockout_d_id_line_6_13_cc035) -> id_line_6_13/1
  id_line_4_9/1 -> d_iq_line_4_9_block/1(State_id_line_4_9_5fb10), id_bus_4_block/6(State_id_line_4_9_61110), id_bus_9_block/2(State_id_line_4_9_8b9da)
  iq_line_7_9/1 -> d_id_line_7_9_block/1(State_iq_line_7_9_66432), iq_bus_9_block/3(State_iq_line_7_9_360e6), iq_bus_7_block/3(State_iq_line_7_9_fd2c4)
  iq_line_3_4/1 -> d_id_line_3_4_block/2(State_iq_line_3_4_6988a), d_iq_line_3_4_block/2(State_iq_line_3_4_fc92d), iq_bus_3_block/4(State_iq_line_3_4_658ee), iq_bus_4_block/3(State_iq_line_3_4_962a3)
  iq_line_14_18/1 -> d_id_line_14_18_block/2(State_iq_line_14_18_a74d0), d_iq_line_14_18_block/2(State_iq_line_14_18_dd432), iq_bus_14_block/4(State_iq_line_14_18_e379d), iq_bus_18_block/2(State_iq_line_14_18_2108f)
  d_iq_line_5_6_block/1(Blockout_d_iq_line_5_6_9d95c) -> iq_line_5_6/1
  iq_line_9_14/1 -> d_iq_line_9_14_block/2(State_iq_line_9_14_07292), iq_bus_14_block/2(State_iq_line_9_14_48c7f), iq_bus_9_block/5(State_iq_line_9_14_10f53), d_id_line_9_14_block/2(State_iq_line_9_14_72453)
  d_vq_bus_3_block/1(Blockout_d_vq_bus_3_9f56f) -> vq_bus_3/1
  d_id_line_5_6_block/1(Blockout_d_id_line_5_6_7c54f) -> id_line_5_6/1
  d_iq_load_13_block/1(Blockout_d_iq_load_13_714c3) -> iq_load_13/1
  id_load_13/1 -> id_bus_13_block/1(State_id_load_13_0fa38), d_id_load_13_block/1(State_id_load_13_999eb), d_iq_load_13_block/1(State_id_load_13_29b8c)
  vq_bus_7/1 -> d_iq_line_7_9_block/2(State_vq_bus_7_de92f), d_iq_line_4_7_block/3(State_vq_bus_7_17236), d_vd_bus_7_block/2(State_vq_bus_7_3c6fe), d_iq_line_7_8_block/2(State_vq_bus_7_4632e)
  d_id_line_4_9_block/1(Blockout_d_id_line_4_9_c5562) -> id_line_4_9/1
  iq_load_13/1 -> d_id_load_13_block/2(State_iq_load_13_edcc2), iq_bus_13_block/1(State_iq_load_13_3bbcd), d_iq_load_13_block/2(State_iq_load_13_dc329)
  d_id_line_4_7_block/1(Blockout_d_id_line_4_7_734b6) -> id_line_4_7/1
  id_line_7_9/1 -> d_iq_line_7_9_block/1(State_id_line_7_9_a5037), id_bus_9_block/3(State_id_line_7_9_16065), id_bus_7_block/3(State_id_line_7_9_11a60)
  vd_bus_12/1 -> d_vq_bus_12_block/2(State_vd_bus_12_1eb7a), d_id_line_12_16_block/3(State_vd_bus_12_7f21e), d_id_line_6_12_block/3(State_vd_bus_12_ff782), d_id_line_12_13_block/3(State_vd_bus_12_5b3a8), d_id_load_12_block/3(State_vd_bus_12_f1be8)
  iq_load_14/1 -> d_iq_load_14_block/2(State_iq_load_14_ef373), iq_bus_14_block/1(State_iq_load_14_41c2f), d_id_load_14_block/2(State_iq_load_14_2d6b8)
  id_load_3/1 -> id_bus_3_block/2(State_id_load_3_b4943), d_iq_load_3_block/1(State_id_load_3_d79a9), d_id_load_3_block/1(State_id_load_3_166da)
  d_id_line_12_16_block/1(Blockout_d_id_line_12_16_c0fbf) -> id_line_12_16/1
  vq_bus_13/1 -> d_vd_bus_13_block/2(State_vq_bus_13_424b0), d_iq_line_13_14_block/3(State_vq_bus_13_82621), d_iq_load_13_block/3(State_vq_bus_13_7eda7), d_iq_line_6_13_block/3(State_vq_bus_13_5730a), d_iq_line_13_17_block/3(State_vq_bus_13_d3788), d_iq_line_12_13_block/4(State_vq_bus_13_52e4e)
  d_id_line_2_4_block/1(Blockout_d_id_line_2_4_3a4a6) -> id_line_2_4/1
  d_iq_line_4_7_block/1(Blockout_d_iq_line_4_7_8270d) -> iq_line_4_7/1
  d_iq_load_11_block/1(Blockout_d_iq_load_11_90745) -> iq_load_11/1
  iq_load_6/1 -> iq_bus_6_block/2(State_iq_load_6_74227), d_iq_load_6_block/2(State_iq_load_6_40498), d_id_load_6_block/2(State_iq_load_6_5ea6c)
  d_id_load_6_block/1(Blockout_d_id_load_6_d0eb4) -> id_load_6/1
  d_vq_bus_1_block/1(Blockout_d_vq_bus_1_ae37f) -> vq_bus_1/1
  d_iq_load_5_block/1(Blockout_d_iq_load_5_ab2ba) -> iq_load_5/1
  vq_bus_10/1 -> d_vd_bus_10_block/2(State_vq_bus_10_6f6de), d_iq_line_10_11_block/3(State_vq_bus_10_f1a56), d_iq_line_9_10_block/3(State_vq_bus_10_aebb4), d_iq_load_10_block/3(State_vq_bus_10_81f02)
  iq_line_13_14/1 -> d_id_line_13_14_block/2(State_iq_line_13_14_4cdf7), d_iq_line_13_14_block/2(State_iq_line_13_14_4a60c), iq_bus_13_block/4(State_iq_line_13_14_1f5ac), iq_bus_14_block/3(State_iq_line_13_14_26ead)
  iq_line_1_5/1 -> d_id_line_1_5_block/2(State_iq_line_1_5_368c4), iq_bus_1_block/3(State_iq_line_1_5_234de), iq_bus_5_block/2(State_iq_line_1_5_5a6f8), d_iq_line_1_5_block/2(State_iq_line_1_5_cd4fe)
  d_id_load_5_block/1(Blockout_d_id_load_5_99e2f) -> id_load_5/1
  id_load_2/1 -> d_id_load_2_block/1(State_id_load_2_f170a), id_bus_2_block/2(State_id_load_2_24351), d_iq_load_2_block/1(State_id_load_2_e4c0e)
  d_vd_bus_17_block/1(Blockout_d_vd_bus_17_dc311) -> vd_bus_17/1
  d_vd_bus_16_block/1(Blockout_d_vd_bus_16_67f66) -> vd_bus_16/1
  id_load_11/1 -> d_id_load_11_block/1(State_id_load_11_628b0), id_bus_11_block/1(State_id_load_11_85329), d_iq_load_11_block/1(State_id_load_11_9ab2f)
  d_vq_bus_14_block/1(Blockout_d_vq_bus_14_55ab8) -> vq_bus_14/1
  vq_bus_5/1 -> d_iq_line_5_6_block/2(State_vq_bus_5_491c0), d_iq_load_5_block/3(State_vq_bus_5_cfb62), d_iq_line_1_5_block/4(State_vq_bus_5_25d28), d_iq_line_2_5_block/4(State_vq_bus_5_3bd85), d_iq_line_4_5_block/4(State_vq_bus_5_79571), d_vd_bus_5_block/2(State_vq_bus_5_bfac5)
  d_vd_bus_13_block/1(Blockout_d_vd_bus_13_9076d) -> vd_bus_13/1
  id_load_14/1 -> d_id_load_14_block/1(State_id_load_14_2e0ae), id_bus_14_block/1(State_id_load_14_1cf8a), d_iq_load_14_block/1(State_id_load_14_07147)
  vd_bus_9/1 -> d_id_load_9_block/3(State_vd_bus_9_e4c71), d_id_line_7_9_block/3(State_vd_bus_9_0bd7a), d_id_line_9_14_block/4(State_vd_bus_9_8eb23), d_id_line_4_9_block/3(State_vd_bus_9_e9340), d_id_line_9_10_block/4(State_vd_bus_9_919cb), d_vq_bus_9_block/2(State_vd_bus_9_ab45c)
  iq_load_12/1 -> d_iq_load_12_block/2(State_iq_load_12_acbdc), iq_bus_12_block/1(State_iq_load_12_82e1a), d_id_load_12_block/2(State_iq_load_12_84390)
  iq_load_3/1 -> d_iq_load_3_block/2(State_iq_load_3_276a1), iq_bus_3_block/2(State_iq_load_3_1a588), d_id_load_3_block/2(State_iq_load_3_14c81)
  d_vd_bus_3_block/1(Blockout_d_vd_bus_3_5883d) -> vd_bus_3/1
  d_vq_bus_2_block/1(Blockout_d_vq_bus_2_5ca2e) -> vq_bus_2/1
  iq_line_2_4/1 -> d_iq_line_2_4_block/2(State_iq_line_2_4_af312), iq_bus_2_block/5(State_iq_line_2_4_78218), iq_bus_4_block/2(State_iq_line_2_4_9abf1), d_id_line_2_4_block/2(State_iq_line_2_4_3e60f)
  vd_bus_5/1 -> d_vq_bus_5_block/2(State_vd_bus_5_1cd26), d_id_line_1_5_block/4(State_vd_bus_5_58650), d_id_line_2_5_block/4(State_vd_bus_5_c8ea7), d_id_line_5_6_block/2(State_vd_bus_5_45df8), d_id_line_4_5_block/4(State_vd_bus_5_24735), d_id_load_5_block/3(State_vd_bus_5_96189)
  id_line_13_17/1 -> d_id_line_13_17_block/1(State_id_line_13_17_86061), id_bus_13_block/5(State_id_line_13_17_1d2fa), id_bus_17_block/2(State_id_line_13_17_58c1b), d_iq_line_13_17_block/1(State_id_line_13_17_62ede)
  iq_load_4/1 -> iq_bus_4_block/1(State_iq_load_4_ce024), d_iq_load_4_block/2(State_iq_load_4_d8cb8), d_id_load_4_block/2(State_iq_load_4_3a649)
  iq_line_1_2/1 -> d_id_line_1_2_block/2(State_iq_line_1_2_aada7), d_iq_line_1_2_block/2(State_iq_line_1_2_a6f16), iq_bus_2_block/3(State_iq_line_1_2_2f4d7), iq_bus_1_block/2(State_iq_line_1_2_a608a)
  vq_bus_8/1 -> d_iq_line_7_8_block/3(State_vq_bus_8_957c7), d_vd_bus_8_block/2(State_vq_bus_8_e0284), vq_bus_8_out_block/1(State_vq_bus_8_b3a86)
  id_line_10_11/1 -> d_id_line_10_11_block/1(State_id_line_10_11_cd03d), id_bus_10_block/3(State_id_line_10_11_6295b), id_bus_11_block/3(State_id_line_10_11_3f962), d_iq_line_10_11_block/1(State_id_line_10_11_672ad)
  iq_line_12_13/1 -> d_id_line_12_13_block/2(State_iq_line_12_13_bd70b), d_iq_line_12_13_block/2(State_iq_line_12_13_eef70), iq_bus_12_block/3(State_iq_line_12_13_b5bd7), iq_bus_13_block/3(State_iq_line_12_13_f5a73)
  id_line_9_14/1 -> id_bus_9_block/5(State_id_line_9_14_00d21), d_id_line_9_14_block/1(State_id_line_9_14_b515e), d_iq_line_9_14_block/1(State_id_line_9_14_dd4a4), id_bus_14_block/2(State_id_line_9_14_3a619)
  vq_bus_11/1 -> d_vd_bus_11_block/2(State_vq_bus_11_98fc3), d_iq_line_6_11_block/3(State_vq_bus_11_5a0e6), d_iq_line_10_11_block/4(State_vq_bus_11_9096b), d_iq_load_11_block/3(State_vq_bus_11_ff375), d_iq_line_11_15_block/3(State_vq_bus_11_fe1e1)
  vq_bus_14/1 -> d_vd_bus_14_block/2(State_vq_bus_14_3a1f7), d_iq_line_9_14_block/3(State_vq_bus_14_753fc), d_iq_line_14_18_block/3(State_vq_bus_14_bc785), d_iq_line_13_14_block/4(State_vq_bus_14_d664c), d_iq_load_14_block/3(State_vq_bus_14_cd634)
  d_iq_line_13_14_block/1(Blockout_d_iq_line_13_14_49b1d) -> iq_line_13_14/1
  id_line_6_12/1 -> id_bus_6_block/5(State_id_line_6_12_d416e), d_iq_line_6_12_block/1(State_id_line_6_12_268a8), id_bus_12_block/2(State_id_line_6_12_49cbb), d_id_line_6_12_block/1(State_id_line_6_12_9e271)
  d_vd_bus_6_block/1(Blockout_d_vd_bus_6_b094f) -> vd_bus_6/1
  id_line_1_2/1 -> d_iq_line_1_2_block/1(State_id_line_1_2_008aa), id_bus_1_block/2(State_id_line_1_2_9da7e), id_bus_2_block/3(State_id_line_1_2_672bc), d_id_line_1_2_block/1(State_id_line_1_2_4e64f)
  id_line_6_11/1 -> id_bus_6_block/4(State_id_line_6_11_01f81), d_id_line_6_11_block/1(State_id_line_6_11_a0eef), d_iq_line_6_11_block/1(State_id_line_6_11_3e498), id_bus_11_block/2(State_id_line_6_11_4f772)
  d_vq_bus_7_block/1(Blockout_d_vq_bus_7_86357) -> vq_bus_7/1
  vq_bus_4/1 -> d_iq_line_4_7_block/2(State_vq_bus_4_757cb), d_iq_line_2_4_block/4(State_vq_bus_4_4a861), d_iq_line_4_5_block/3(State_vq_bus_4_22b10), d_iq_line_4_9_block/2(State_vq_bus_4_2d444), d_vd_bus_4_block/2(State_vq_bus_4_a1d9b), d_iq_load_4_block/3(State_vq_bus_4_a0870), d_iq_line_3_4_block/4(State_vq_bus_4_4eaa9)
  vd_bus_18/1 -> d_vq_bus_18_block/2(State_vd_bus_18_940ad), vd_bus_18_out_block/1(State_vd_bus_18_46c9f), d_id_line_14_18_block/4(State_vd_bus_18_b444f)
  d_id_load_13_block/1(Blockout_d_id_load_13_e8012) -> id_load_13/1
  id_line_5_6/1 -> d_iq_line_5_6_block/1(State_id_line_5_6_8d92b), id_bus_5_block/5(State_id_line_5_6_d193e), id_bus_6_block/3(State_id_line_5_6_cecb9)
  d_vq_bus_18_block/1(Blockout_d_vq_bus_18_9e140) -> vq_bus_18/1
  id_line_4_7/1 -> d_iq_line_4_7_block/1(State_id_line_4_7_b85c3), id_bus_4_block/5(State_id_line_4_7_02fe7), id_bus_7_block/1(State_id_line_4_7_887cf)
  id_line_4_5/1 -> id_bus_4_block/4(State_id_line_4_5_4eaac), id_bus_5_block/4(State_id_line_4_5_5de68), d_id_line_4_5_block/1(State_id_line_4_5_a3d02), d_iq_line_4_5_block/1(State_id_line_4_5_b6bf8)
  id_load_4/1 -> id_bus_4_block/1(State_id_load_4_4d084), d_id_load_4_block/1(State_id_load_4_9125b), d_iq_load_4_block/1(State_id_load_4_3f12c)
  iq_load_10/1 -> d_id_load_10_block/2(State_iq_load_10_87559), d_iq_load_10_block/2(State_iq_load_10_0f9f7), iq_bus_10_block/1(State_iq_load_10_2ce70)
  id_line_1_5/1 -> id_bus_5_block/2(State_id_line_1_5_464f3), d_id_line_1_5_block/1(State_id_line_1_5_7d5d3), d_iq_line_1_5_block/1(State_id_line_1_5_6753b), id_bus_1_block/3(State_id_line_1_5_b6c3a)
  id_load_6/1 -> id_bus_6_block/2(State_id_load_6_c7fc2), d_id_load_6_block/1(State_id_load_6_6a8f0), d_iq_load_6_block/1(State_id_load_6_8bda4)
  id_load_12/1 -> d_id_load_12_block/1(State_id_load_12_be97f), d_iq_load_12_block/1(State_id_load_12_0975f), id_bus_12_block/1(State_id_load_12_a6028)
  vd_bus_15/1 -> d_vq_bus_15_block/2(State_vd_bus_15_ac75c), d_id_line_11_15_block/4(State_vd_bus_15_a703b), vd_bus_15_out_block/1(State_vd_bus_15_8a646)
  vq_bus_6/1 -> d_vd_bus_6_block/2(State_vq_bus_6_681db), d_iq_line_5_6_block/3(State_vq_bus_6_39104), d_iq_load_6_block/3(State_vq_bus_6_34215), d_iq_line_6_11_block/4(State_vq_bus_6_fa1ab), d_iq_line_6_12_block/4(State_vq_bus_6_e763a), d_iq_line_6_13_block/4(State_vq_bus_6_f0e31), vq_bus_6_out_block/1(State_vq_bus_6_b99ed)
  vd_bus_2/1 -> d_vq_bus_2_block/2(State_vd_bus_2_6d7a2), d_id_load_2_block/3(State_vd_bus_2_22b83), d_id_line_1_2_block/4(State_vd_bus_2_c09e1), d_id_line_2_3_block/3(State_vd_bus_2_5855d), d_id_line_2_4_block/3(State_vd_bus_2_934b9), d_id_line_2_5_block/3(State_vd_bus_2_cba5a), vd_bus_2_out_block/1(State_vd_bus_2_3f94d)
  d_iq_line_1_5_block/1(Blockout_d_iq_line_1_5_d4afd) -> iq_line_1_5/1
  d_iq_line_7_9_block/1(Blockout_d_iq_line_7_9_01bdc) -> iq_line_7_9/1
  d_iq_line_13_17_block/1(Blockout_d_iq_line_13_17_2fa46) -> iq_line_13_17/1
  d_vq_bus_17_block/1(Blockout_d_vq_bus_17_6d857) -> vq_bus_17/1
  d_iq_line_2_5_block/1(Blockout_d_iq_line_2_5_1f062) -> iq_line_2_5/1
  d_iq_line_9_10_block/1(Blockout_d_iq_line_9_10_9f0b6) -> iq_line_9_10/1
  d_id_line_11_15_block/1(Blockout_d_id_line_11_15_7b448) -> id_line_11_15/1
  d_id_line_2_3_block/1(Blockout_d_id_line_2_3_6d07a) -> id_line_2_3/1
  d_iq_load_14_block/1(Blockout_d_iq_load_14_aff57) -> iq_load_14/1
  d_iq_load_4_block/1(Blockout_d_iq_load_4_a1a6f) -> iq_load_4/1
  d_id_line_12_13_block/1(Blockout_d_id_line_12_13_a63f9) -> id_line_12_13/1
  d_id_line_13_14_block/1(Blockout_d_id_line_13_14_fab77) -> id_line_13_14/1
  d_iq_line_14_18_block/1(Blockout_d_iq_line_14_18_2b84d) -> iq_line_14_18/1
  d_id_line_1_5_block/1(Blockout_d_id_line_1_5_95dd5) -> id_line_1_5/1
  d_id_line_3_4_block/1(Blockout_d_id_line_3_4_73a35) -> id_line_3_4/1
  d_id_line_4_5_block/1(Blockout_d_id_line_4_5_bb2ec) -> id_line_4_5/1
  d_iq_line_6_12_block/1(Blockout_d_iq_line_6_12_bda61) -> iq_line_6_12/1
  d_id_line_6_11_block/1(Blockout_d_id_line_6_11_26563) -> id_line_6_11/1
  d_iq_line_2_4_block/1(Blockout_d_iq_line_2_4_8ffa8) -> iq_line_2_4/1
  d_id_load_10_block/1(Blockout_d_id_load_10_a8029) -> id_load_10/1
  d_vq_bus_16_block/1(Blockout_d_vq_bus_16_4b2eb) -> vq_bus_16/1
  d_vd_bus_2_block/1(Blockout_d_vd_bus_2_7ca8e) -> vd_bus_2/1
  d_iq_load_6_block/1(Blockout_d_iq_load_6_d9bfd) -> iq_load_6/1
  d_vq_bus_10_block/1(Blockout_d_vq_bus_10_bbdbe) -> vq_bus_10/1
  d_vq_bus_13_block/1(Blockout_d_vq_bus_13_eb8c6) -> vq_bus_13/1
  d_iq_line_2_3_block/1(Blockout_d_iq_line_2_3_79888) -> iq_line_2_3/1
  d_id_load_2_block/1(Blockout_d_id_load_2_a876e) -> id_load_2/1
  d_iq_line_1_2_block/1(Blockout_d_iq_line_1_2_8e65d) -> iq_line_1_2/1
  d_id_load_4_block/1(Blockout_d_id_load_4_eca8f) -> id_load_4/1
  d_id_load_9_block/1(Blockout_d_id_load_9_e6f54) -> id_load_9/1
  d_iq_line_12_13_block/1(Blockout_d_iq_line_12_13_64197) -> iq_line_12_13/1
  d_iq_line_4_9_block/1(Blockout_d_iq_line_4_9_8879d) -> iq_line_4_9/1
  d_iq_line_6_13_block/1(Blockout_d_iq_line_6_13_6bd96) -> iq_line_6_13/1
  d_iq_load_3_block/1(Blockout_d_iq_load_3_49ef1) -> iq_load_3/1
  d_iq_line_9_14_block/1(Blockout_d_iq_line_9_14_f1895) -> iq_line_9_14/1
  d_iq_load_10_block/1(Blockout_d_iq_load_10_8a684) -> iq_load_10/1
  d_vd_bus_10_block/1(Blockout_d_vd_bus_10_484a7) -> vd_bus_10/1
  d_vd_bus_11_block/1(Blockout_d_vd_bus_11_0b5d5) -> vd_bus_11/1
  d_vd_bus_12_block/1(Blockout_d_vd_bus_12_63d51) -> vd_bus_12/1
  d_vd_bus_14_block/1(Blockout_d_vd_bus_14_7c236) -> vd_bus_14/1
  d_vd_bus_15_block/1(Blockout_d_vd_bus_15_6b2d1) -> vd_bus_15/1
  d_vd_bus_1_block/1(Blockout_d_vd_bus_1_52715) -> vd_bus_1/1
  d_vd_bus_4_block/1(Blockout_d_vd_bus_4_c11bd) -> vd_bus_4/1
  d_vd_bus_5_block/1(Blockout_d_vd_bus_5_c33ea) -> vd_bus_5/1
  d_vd_bus_8_block/1(Blockout_d_vd_bus_8_50ae4) -> vd_bus_8/1
  d_vd_bus_9_block/1(Blockout_d_vd_bus_9_6a7a4) -> vd_bus_9/1
  d_vq_bus_5_block/1(Blockout_d_vq_bus_5_be7b6) -> vq_bus_5/1
  d_vq_bus_6_block/1(Blockout_d_vq_bus_6_55bf0) -> vq_bus_6/1
  d_vq_bus_8_block/1(Blockout_d_vq_bus_8_795e4) -> vq_bus_8/1
  d_vq_bus_9_block/1(Blockout_d_vq_bus_9_d5b49) -> vq_bus_9/1
